simulink model "CAN"  (R2018b)
settings: Solver=FixedStepDiscrete  StartTime=0.0  StopTime=10.0  RelTol=1e-3
undefined symbols (not defined in the file): canChannel, CR, LF, serial
libraries: canfdlib x4, canfdmsglib x2, instrumentlib x2
settings Model: Creator=Alex  LastModifiedBy=Alex

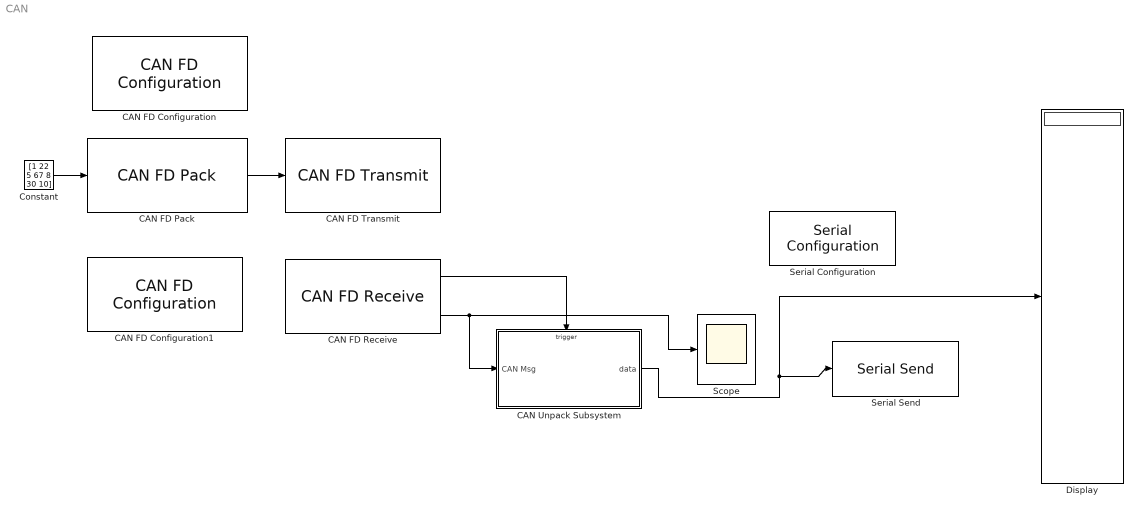
== system CAN ==
  CAN FD Configuration : canfdlib/CAN FD Configuration  Device=Vector Virtual 1 (Channel 1)  ObjConstructor=canChannel('Vector', 'Virtual 1', 1, 'ProtocolMode', 'CAN FD')  ArbitrationBusSpeed=1000000  ArbitrationSJW=2  ArbitrationTSEG1=6  ArbitrationTSEG2=3  DataBusSpeed=8000000  DataSJW=2  DataTSEG1=6  DataTSEG2=3  BusFrequency=20  ArbitrationPrescaler=5  DataPrescaler=2  AckMode=Normal  BlockHandle=4.0002
      settings: SourceProductName=Vehicle Network Toolbox  SourceProductBaseCode=VN
  CAN FD Configuration1 : canfdlib/CAN FD Configuration  Device=Vector Virtual 1 (Channel 2)  ObjConstructor=canChannel('Vector', 'Virtual 1', 2, 'ProtocolMode', 'CAN FD')  ArbitrationBusSpeed=1000000  ArbitrationSJW=2  ArbitrationTSEG1=6  ArbitrationTSEG2=3  DataBusSpeed=8000000  DataSJW=2  DataTSEG1=6  DataTSEG2=3  BusFrequency=20  ArbitrationPrescaler=5  DataPrescaler=2  AckMode=Normal  BlockHandle=5.0002
      settings: SourceProductName=Vehicle Network Toolbox  SourceProductBaseCode=VN
  CAN FD Pack : canfdmsglib/CAN FD Pack  MsgList=(none)  MsgName=Msg  ProtocolMode=CAN FD  MsgIDType=Standard (11-bit identifier)  MsgIdentifier=500  MsgLength=8  NSignals=0  StartBits=0  SignalSizes=0  ByteOrders=0  DataTypes=0  MultiplexTypes=0  MultiplexValues=0  Factors=0  Offsets=0  Minimums=0  Maximums=0  Remote=off  ApplyMinMax=off  BRSSwitch=off
      settings: SourceProductName=Simulink Real-Time  DataFormat=raw data
  CAN FD Receive : canfdlib/CAN FD Receive  BlockHandle=7.0002  Device=Vector Virtual 1 (Channel 2)  ObjConstructor=canChannel('Vector', 'Virtual 1', 2, 'ProtocolMode', 'CAN FD')  EnableStandardIDsFilter=off  StandardIDs=0  EnableExtendedIDsFilter=off  ExtendedIDs=0  SampleTime=0.01  MsgsPerTimestep=all  StdIDsCombo=Allow all  ExtIDsCombo=Allow all  InternalFilterUpdateStatus=on
      settings: SourceProductName=Vehicle Network Toolbox  SourceProductBaseCode=VN
  CAN FD Transmit : canfdlib/CAN FD Transmit  BlockHandle=8.0002  Device=Vector Virtual 1 (Channel 1)  ObjConstructor=canChannel('Vector', 'Virtual 1', 1, 'ProtocolMode', 'CAN FD')  EnablePeriodicTransmit=off  MessagePeriod=2
      settings: SourceProductName=Vehicle Network Toolbox  SourceProductBaseCode=VN
  CAN Unpack Subsystem : Subsystem  TreatAsAtomicUnit=on
  Constant : Constant  Value=[1 22 5 67 8 30 10]  OutDataTypeStr=uint8  SampleTime=1
  Display : Display
  Scope : Scope
  Serial Configuration : instrumentlib/Serial Configuration  Priority=-200000  ComPortMenu=COM5  ComPort=COM5  ObjConstructor=serial('COM5');  BaudRate=9600  DataBits=8  Parity=none  StopBits=1  FlowControl=none  Timeout=10  ByteOrder=LittleEndian
  Serial Send : instrumentlib/Serial Send  ComPortMenu=COM5  ComPort=COM5  ObjConstructor=serial('COM5');  Terminator=CR/LF ('\r\n')  EnableBlockingMode=on
  wires:
  Constant/1 -> CAN FD Pack/1
  CAN FD Pack/1 -> CAN FD Transmit/1
  CAN FD Receive/2 -> Scope/1, CAN Unpack Subsystem/1(CAN Msg)
  CAN Unpack Subsystem/1(data) -> Serial Send/1, Display/1
  CAN FD Receive/1 -> CAN Unpack Subsystem/Trigger

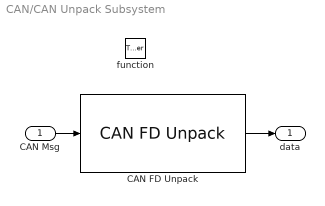
== system CAN/CAN Unpack Subsystem ==
  CAN Msg : Inport
  function : TriggerPort  TriggerType=function-call  VariantControl=Variant
  CAN FD Unpack : canfdmsglib/CAN FD Unpack  MsgList=(none)  MsgName=Msg  ProtocolMode=CAN FD  MsgIDType=Standard (11-bit identifier)  MsgIdentifier=500  MsgLength=8  NSignals=0  IDPort=off  TimestampPort=off  ErrorPort=off  RemotePort=off  LengthPort=off  StatusPort=off  BRSPort=off  ESIPort=off  DLCPort=off  StartBits=0  SignalSizes=0  ByteOrders=0  DataTypes=0  MultiplexTypes=0  MultiplexValues=0  Factors=0  Offsets=0  Minimums=0  Maximums=0  ApplyMinMax=off
      settings: SourceProductName=Simulink Real-Time  DataFormat=raw data
  data : Outport
  wires:
  CAN Msg/1 -> CAN FD Unpack/1
  CAN FD Unpack/1 -> data/1
